simulink model "lab6"  (R2022b)
settings: Solver=VariableStepAuto  StartTime=0.0  StopTime=10.0  RelTol=1e-3
undefined symbols (not defined in the file or in its folder): a, v
libraries: cstblocks x1
settings Model: Creator=S270874  LastModifiedBy=franc
settings ModelReferenceCC: EnableRefExpFcnMdlSchedulingChecks=on

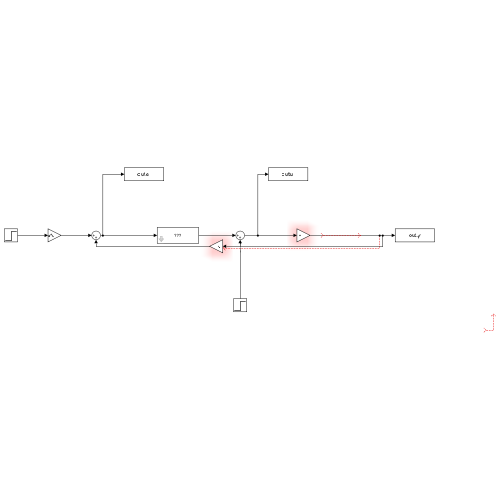
[thumbnail: Simulink's stored preview of the top-level diagram]
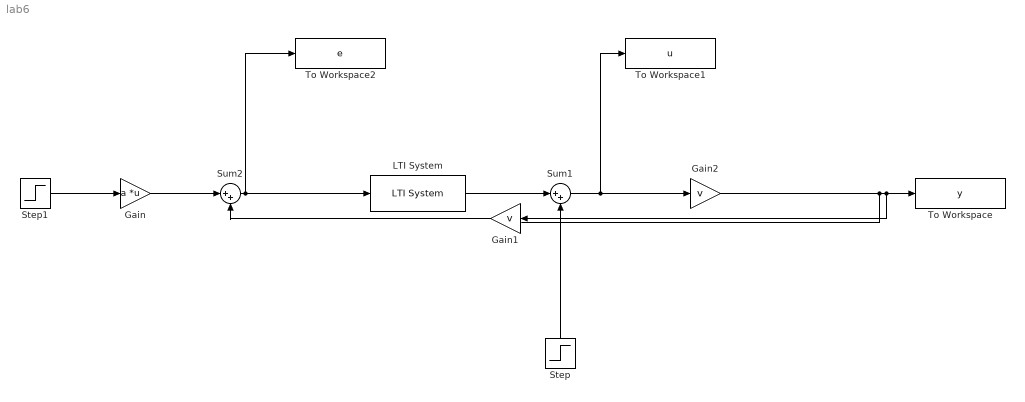
== system lab6 ==
  Gain : Gain  Gain=a  Multiplication=Matrix(K*u)
  Gain1 : Gain  Gain=v
  Gain2 : Gain  Gain=v
  LTI System : cstblocks/LTI System  sys=sys_x  IC=[]
  Step : Step  Time=0  SampleTime=0
  Step1 : Step  Time=0  SampleTime=0
  Sum1 : Sum  Inputs=|++
  Sum2 : Sum  Inputs=|++
  To Workspace : ToWorkspace  VariableName=y  SaveFormat=Timeseries  SampleTime=-1
  To Workspace1 : ToWorkspace  VariableName=u  SaveFormat=Timeseries  SampleTime=-1
  To Workspace2 : ToWorkspace  VariableName=e  SaveFormat=Timeseries  SampleTime=-1
  wires:
  ? -> ?
  Step1/1 -> Gain/1
  Step/1 -> Sum1/2
  Sum1/1 -> Gain2/1, To Workspace1/1
  LTI System/1 -> Sum1/1
  Sum2/1 -> To Workspace2/1, LTI System/1
  ? -> ?
  Gain2/1 -> Gain1/1, To Workspace/1
  Gain/1 -> Sum2/1
  Gain1/1 -> Sum2/2
